simulink model "fuzzypid"  (R2021a)
settings: Solver=VariableStepAuto  StartTime=0.0  StopTime=1  RelTol=1e-3
libraries: fuzblock x1
settings Model: Creator=Sirius  LastModifiedBy=Sirius

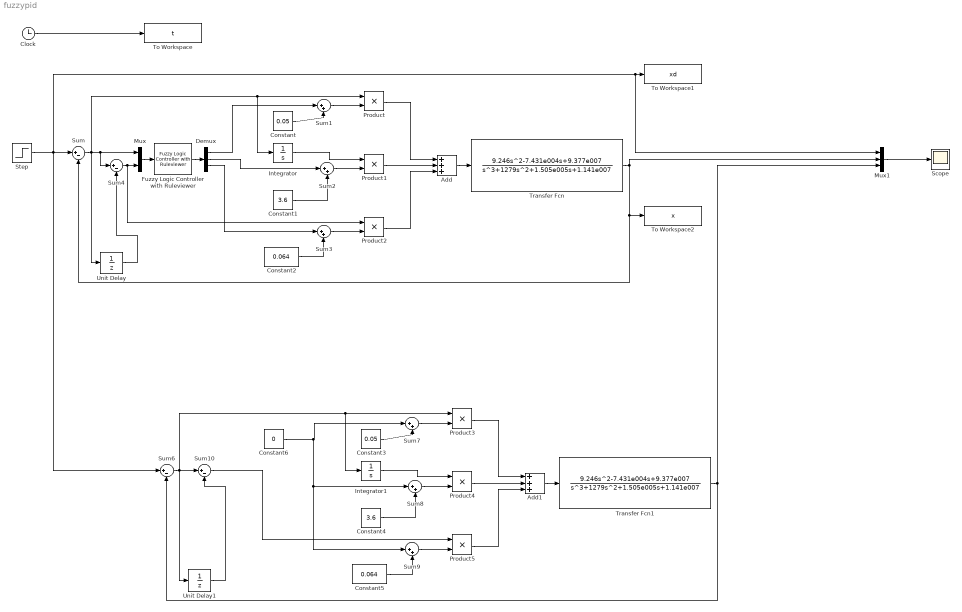
== system fuzzypid ==
  Add : Sum  Inputs=+++
  Add1 : Sum  Inputs=+++
  Clock : Clock
  Constant : Constant  Value=0.05
  Constant1 : Constant  Value=3.6
  Constant2 : Constant  Value=0.064
  Constant3 : Constant  Value=0.05
  Constant4 : Constant  Value=3.6
  Constant5 : Constant  Value=0.064
  Constant6 : Constant  Value=0
  Demux : Demux  Outputs=3
  Fuzzy Logic Controller with Ruleviewer : fuzblock/Fuzzy Logic  Controller  with Ruleviewer  fismatrix=pid  Ts=0.01
  Integrator : Integrator
  Integrator1 : Integrator
  Mux : Mux  Inputs=2
  Mux1 : Mux  Inputs=3
  Product{,1..5} (6 alike) : Product
  Scope : Scope
  Step : Step  Time=0  SampleTime=0
  Sum{,4,6,10} (4 alike) : Sum  Inputs=|+-
  Sum{1..3,7..9} (6 alike) : Sum  Inputs=|++
  To Workspace : ToWorkspace  VariableName=t  SaveFormat=Timeseries  SampleTime=-1
  To Workspace1 : ToWorkspace  VariableName=xd  SaveFormat=Timeseries  SampleTime=-1
  To Workspace2 : ToWorkspace  VariableName=x  SaveFormat=Timeseries  SampleTime=-1
  Transfer Fcn : TransferFcn  Numerator=[9.246 -7.431e004 9.377e007]  Denominator=[1 1279 1.505e005 1.141e007]
  Transfer Fcn1 : TransferFcn  Numerator=[9.246 -7.431e004 9.377e007]  Denominator=[1 1279 1.505e005 1.141e007]
  Unit Delay : UnitDelay  SampleTime=-1  HasFrameUpgradeWarning=on
  Unit Delay1 : UnitDelay  SampleTime=-1  HasFrameUpgradeWarning=on
  wires:
  Clock/1 -> To Workspace/1
  Product/1 -> Add/1
  Product1/1 -> Add/2
  Product2/1 -> Add/3
  Integrator/1 -> Product1/1
  Add/1 -> Transfer Fcn/1
  Transfer Fcn/1 -> Mux1/2, To Workspace2/1, Sum/2
  Step/1 -> Sum6/1, Mux1/1, To Workspace1/1, Sum/1
  Sum2/1 -> Product1/2
  Sum3/1 -> Product2/2
  Sum1/1 -> Product/2
  Sum/1 -> Unit Delay/1, Integrator/1, Product/1, Mux/1, Sum4/1
  Sum4/1 -> Mux/2, Product2/1
  Constant/1 -> Sum1/2
  Constant1/1 -> Sum2/2
  Constant2/1 -> Sum3/2
  Mux1/1 -> Scope/1
  Fuzzy Logic Controller with Ruleviewer/1 -> Demux/1
  Demux/1 -> Sum1/1
  Demux/2 -> Sum2/1
  Demux/3 -> Sum3/1
  Mux/1 -> Fuzzy Logic Controller with Ruleviewer/1
  Unit Delay/1 -> Sum4/2
  Unit Delay1/1 -> Sum10/2
  Product4/1 -> Add1/2
  Sum7/1 -> Product3/2
  Integrator1/1 -> Product4/1
  Constant5/1 -> Sum9/2
  Add1/1 -> Transfer Fcn1/1
  Sum9/1 -> Product5/2
  Sum8/1 -> Product4/2
  Product3/1 -> Add1/1
  Constant4/1 -> Sum8/2
  Sum10/1 -> Product5/1
  Sum6/1 -> Unit Delay1/1, Integrator1/1, Product3/1, Sum10/1
  Transfer Fcn1/1 -> Mux1/3, Sum6/2
  Constant3/1 -> Sum7/2
  Product5/1 -> Add1/3
  Constant6/1 -> Sum9/1, Sum8/1, Sum7/1
